simulink model "FireFighter_original"  (R2014a)
settings: Solver=ode45  StartTime=0.0  StopTime=150  RelTol=1e-3
undefined symbols (not defined in the file): DiscIntNeverNeededParam, sigbuilder_block
libraries: simulink x68
(part 3 of 6)

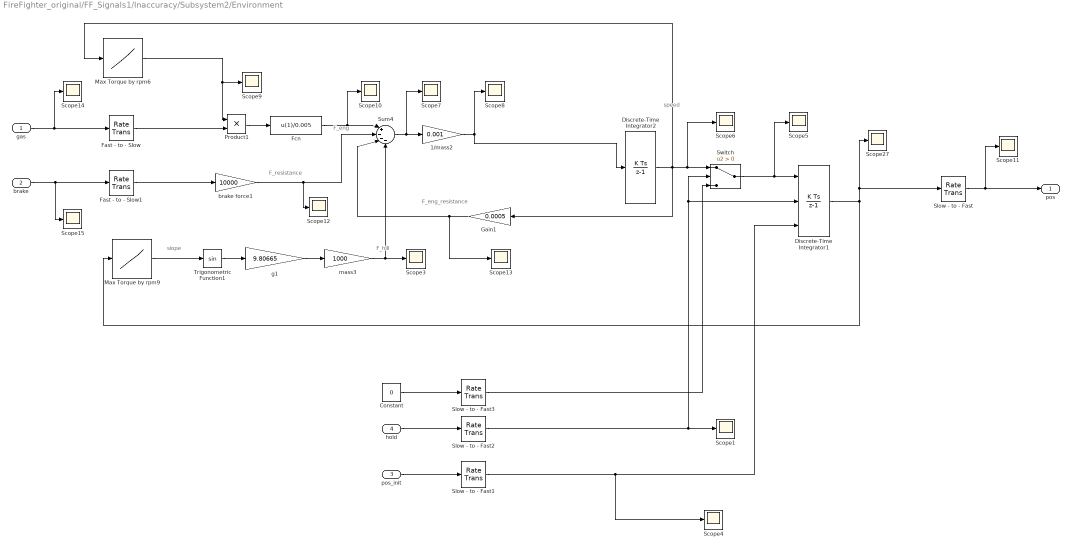
== system FireFighter_original/FF_Signals1/Inaccuracy/Subsystem2/Environment ==
  note: F_hill
  note: F_eng_resistance
  note: F_resistance
  note: F_eng
  note: speed
  note: slope
  gas : Inport
  brake : Inport  Port=2
  pos_init : Inport  Port=3
  hold : Inport  Port=4
  1/mass2 : Gain  Gain=0.001
  Constant : Constant  Value=0
  Discrete-Time Integrator1 : DiscreteIntegrator  ExternalReset=rising  InitialConditionSource=external  SampleTime=-1  ICPrevOutput=DiscIntNeverNeededParam  ICPrevScaledInput=DiscIntNeverNeededParam
  Discrete-Time Integrator2 : DiscreteIntegrator  SampleTime=-1  ICPrevOutput=DiscIntNeverNeededParam  ICPrevScaledInput=DiscIntNeverNeededParam
  Fast - to - Slow : RateTransition  OutPortSampleTimeMultiple=0.05  OutPortSampleTime=0.1
  "Fast - to - Slow1 " : RateTransition  OutPortSampleTimeMultiple=0.05  OutPortSampleTime=0.1
  Fcn : Fcn  Expr=u(1)/0.005
  Gain1 : Gain  Gain=0.0005
  Max Torque by rpm6 : Lookup_n-D  NumberOfTableDimensions=1  BreakpointsForDimension1=[0;8;20;28;40;60;80;100;120;140;160;180;200]  Table=[165;180;180;170;170;150;115;97;80;70;60;50;40]  RndMeth=Simplest  InputSameDT=on
  Max Torque by rpm9 : Lookup_n-D  NumberOfTableDimensions=1  BreakpointsForDimension1=[0:1000:15000]  Table=[0;pi/60;pi/30;pi/20;pi/15;pi/12;0;0;-pi/18;-pi/36;0;0;0;0;0;0]  RndMeth=Simplest  InputSameDT=on
  Product1 : Product  RndMeth=Zero
  Scope{1,3..15,27} (15 alike) : Scope
      Scope1 settings: TimeRange=10  YMin=-50  YMax=300  SaveName=ScopeData3
      Scope10 settings: SaveName=ScopeData23
      Scope11 settings: TimeRange=10  YMin=-50  YMax=300  SaveName=ScopeData26
      Scope12 settings: SaveName=ScopeData32
      Scope13 settings: SaveName=ScopeData33
      Scope14 settings: SaveName=ScopeData15
      Scope15 settings: SaveName=ScopeData19
      Scope27 settings: TimeRange=10  YMin=2000  YMax=3600  SaveName=ScopeData49
      Scope3 settings: SaveName=ScopeData8
      Scope4 settings: TimeRange=10  YMin=-50  YMax=300  SaveName=ScopeData13
      Scope5 settings: TimeRange=10  YMin=-50  YMax=300  SaveName=ScopeData50
      Scope6 settings: TimeRange=100  YMin=89.9904  YMax=89.9913  SaveName=ScopeData16
      Scope7 settings: SaveName=ScopeData10
      Scope8 settings: SaveName=ScopeData21
      Scope9 settings: SaveName=ScopeData22
  Slow - to - Fast{,1..3} (4 alike) : RateTransition  OutPortSampleTimeMultiple=0.05  OutPortSampleTime=0.05
  Sum4 : Sum  Inputs=|+---
  Switch : Switch  Criteria=u2 > Threshold
  Trigonometric Function1 : Trigonometry
  brake force1 : Gain  Gain=10000
  g1 : Gain  Gain=9.80665
  mass3 : Gain  Gain=1000
  pos : Outport
  wires:
  Product1/1 -> Fcn/1
  brake force1/1 -> Scope12/1, Sum4/2
  Sum4/1 -> Scope7/1, 1/mass2/1
  Gain1/1 -> Sum4/3, Scope13/1
  gas/1 -> Scope14/1, Fast - to - Slow/1
  brake/1 -> Scope15/1, "Fast - to - Slow1 "/1
  Discrete-Time Integrator2/1 -> Max Torque by rpm6/1, Scope6/1, Switch/1, Gain1/1
  Max Torque by rpm9/1 -> Trigonometric Function1/1
  g1/1 -> mass3/1
  Trigonometric Function1/1 -> g1/1
  mass3/1 -> Sum4/4, Scope3/1
  Fcn/1 -> Scope10/1, Sum4/1
  Fast - to - Slow/1 -> Product1/2
  "Fast - to - Slow1 "/1 -> brake force1/1
  Discrete-Time Integrator1/1 -> Scope27/1, Slow - to - Fast/1, Max Torque by rpm9/1
  Slow - to - Fast/1 -> pos/1, Scope11/1
  Max Torque by rpm6/1 -> Product1/1, Scope9/1
  pos_init/1 -> Slow - to - Fast1/1
  hold/1 -> Slow - to - Fast2/1
  Slow - to - Fast1/1 -> Scope4/1, Discrete-Time Integrator1/3
  Constant/1 -> Slow - to - Fast3/1
  Slow - to - Fast3/1 -> Switch/3
  Switch/1 -> Scope5/1, Discrete-Time Integrator1/1
  Slow - to - Fast2/1 -> Switch/2, Discrete-Time Integrator1/2, Scope1/1
  1/mass2/1 -> Scope8/1, Discrete-Time Integrator2/1

== system FireFighter_original/FF_Signals1/Inaccuracy/Subsystem2/FireFighter ==
  note: current speed
  note: speed=90
  pos : Inport
  Constant : Constant  Value=0
  Constant1 : Constant  Value=0
  Constant2 : Constant  Value=0
  Discrete Derivative : simulink/Discrete/Discrete Derivative  gainval=1.0  ICPrevScaledInput=0.0  InputProcessing=Inherited  OutMin=[]  OutMax=[]  OutDataType=fixdt(1, 16)  OutScaling=2^-10  DoSatur=off
  Discrete PID Controller : simulink/Continuous/PID Controller  Controller=PI  TimeDomain=Discrete-time  SampleTime=-1  IntegratorMethod=Forward Euler  FilterMethod=Forward Euler  Form=Parallel  P=0.05  I=0.000228325  D=0  N=100  InitialConditionSource=internal  InitialConditionForIntegrator=0  InitialConditionForFilter=0  ExternalReset=none  LimitOutput=on  UpperSaturationLimit=1  LowerSaturationLimit=-1  LinearizeAsGain=off  AntiWindupMode=back-calculation  Kb=0.01  TrackingMode=off  Kt=1  PParamMin=[]  PParamMax=[]  IParamMin=[]  IParamMax=[]  DParamMin=[]  DParamMax=[]  NParamMin=[]  NParamMax=[]  KbParamMin=[]  KbParamMax=[]  KtParamMin=[]  KtParamMax=[]  POutMin=[]  POutMax=[]  IOutMin=[]  IOutMax=[]  DOutMin=[]  DOutMax=[]  NOutMin=[]  NOutMax=[]  KbOutMin=[]  KbOutMax=[]  KtOutMin=[]  KtOutMax=[]  IntegratorOutMin=[]  IntegratorOutMax=[]  FilterOutMin=[]  FilterOutMax=[]  SumOutMin=[]  SumOutMax=[]  SumI1OutMin=[]  SumI1OutMax=[]  SumI2OutMin=[]  SumI2OutMax=[]  SumI3OutMin=[]  SumI3OutMax=[]  SumDOutMin=[]  SumDOutMax=[]  SaturationOutMin=[]  SaturationOutMax=[]  IntegratorContinuousStateAttributes=''  IntegratorStateMustResolveToSignalObject=off  IntegratorRTWStateStorageClass=Auto  FilterContinuousStateAttributes=''  FilterStateMustResolveToSignalObject=off  FilterRTWStateStorageClass=Auto
  Discrete PID Controller1 : simulink/Continuous/PID Controller  Controller=PI  TimeDomain=Discrete-time  SampleTime=-1  IntegratorMethod=Forward Euler  FilterMethod=Forward Euler  Form=Parallel  P=0.05  I=0.000228325  D=0  N=100  InitialConditionSource=internal  InitialConditionForIntegrator=0  InitialConditionForFilter=0  ExternalReset=none  LimitOutput=on  UpperSaturationLimit=1  LowerSaturationLimit=-1  LinearizeAsGain=off  AntiWindupMode=back-calculation  Kb=0.01  TrackingMode=off  Kt=1  PParamMin=[]  PParamMax=[]  IParamMin=[]  IParamMax=[]  DParamMin=[]  DParamMax=[]  NParamMin=[]  NParamMax=[]  KbParamMin=[]  KbParamMax=[]  KtParamMin=[]  KtParamMax=[]  POutMin=[]  POutMax=[]  IOutMin=[]  IOutMax=[]  DOutMin=[]  DOutMax=[]  NOutMin=[]  NOutMax=[]  KbOutMin=[]  KbOutMax=[]  KtOutMin=[]  KtOutMax=[]  IntegratorOutMin=[]  IntegratorOutMax=[]  FilterOutMin=[]  FilterOutMax=[]  SumOutMin=[]  SumOutMax=[]  SumI1OutMin=[]  SumI1OutMax=[]  SumI2OutMin=[]  SumI2OutMax=[]  SumI3OutMin=[]  SumI3OutMax=[]  SumDOutMin=[]  SumDOutMax=[]  SaturationOutMin=[]  SaturationOutMax=[]  IntegratorContinuousStateAttributes=''  IntegratorStateMustResolveToSignalObject=off  IntegratorRTWStateStorageClass=Auto  FilterContinuousStateAttributes=''  FilterStateMustResolveToSignalObject=off  FilterRTWStateStorageClass=Auto
  Fast - to -Slow : RateTransition  OutPortSampleTimeMultiple=0.05  OutPortSampleTime=0.1
  Fast - to -Slow1 : RateTransition  OutPortSampleTimeMultiple=0.05  OutPortSampleTime=0.1
  Fast - to -Slow2 : RateTransition  OutPortSampleTimeMultiple=0.05  OutPortSampleTime=0.1
  Gain1 : Gain  Gain=-1
  Scope{1..2,4..9,11..13} (11 alike) : Scope
      Scope1 settings: YMin=-300  YMax=300  SaveName=ScopeData52
      Scope11 settings: YMin=-300  YMax=300  SaveName=ScopeData28
      Scope12 settings: YMin=-300  YMax=300  SaveName=ScopeData30
      Scope13 settings: SaveName=ScopeData31
      Scope2 settings: YMin=-300  YMax=300  SaveName=ScopeData2
      Scope4 settings: YMin=-300  YMax=300  SaveName=ScopeData17
      Scope5 settings: SaveName=ScopeData20
      Scope6 settings: YMin=-300  YMax=300  SaveName=ScopeData18
      Scope7 settings: YMin=-300  YMax=300  SaveName=ScopeData24
      Scope8 settings: TimeRange=10  SaveName=ScopeData25
      Scope9 settings: SaveName=ScopeData38
  Slow - to - Fast : RateTransition  OutPortSampleTimeMultiple=0.05  OutPortSampleTime=0.05
  Slow - to - Fast1 : RateTransition  OutPortSampleTimeMultiple=0.05  OutPortSampleTime=0.05
  Sum : Sum  Inputs=|+-
  Switch : Switch
  Switch1 : Switch
  gas : Outport
  brake : Outport  Port=2
  wires:
  Discrete Derivative/1 -> Scope8/1, Sum/2
  Discrete PID Controller/1 -> Scope2/1, Scope7/1, Switch/1, Switch/2, Switch1/2, Gain1/1
  Gain1/1 -> Switch1/3
  Switch/1 -> Slow - to - Fast/1, Scope4/1
  Constant/1 -> Switch/3, Switch1/1
  Switch1/1 -> Slow - to - Fast1/1, Scope6/1
  pos/1 -> Scope13/1, Fast - to -Slow/1
  Sum/1 -> Discrete PID Controller/1, Scope9/1
  Fast - to -Slow/1 -> Discrete Derivative/1, Scope5/1
  Slow - to - Fast/1 -> Scope11/1, gas/1
  Slow - to - Fast1/1 -> Scope12/1, brake/1
  Constant2/1 -> Fast - to -Slow1/1
  Fast - to -Slow1/1 -> Sum/1
  Discrete PID Controller1/1 -> Scope1/1
  Constant1/1 -> Fast - to -Slow2/1
  Fast - to -Slow2/1 -> Discrete PID Controller1/1

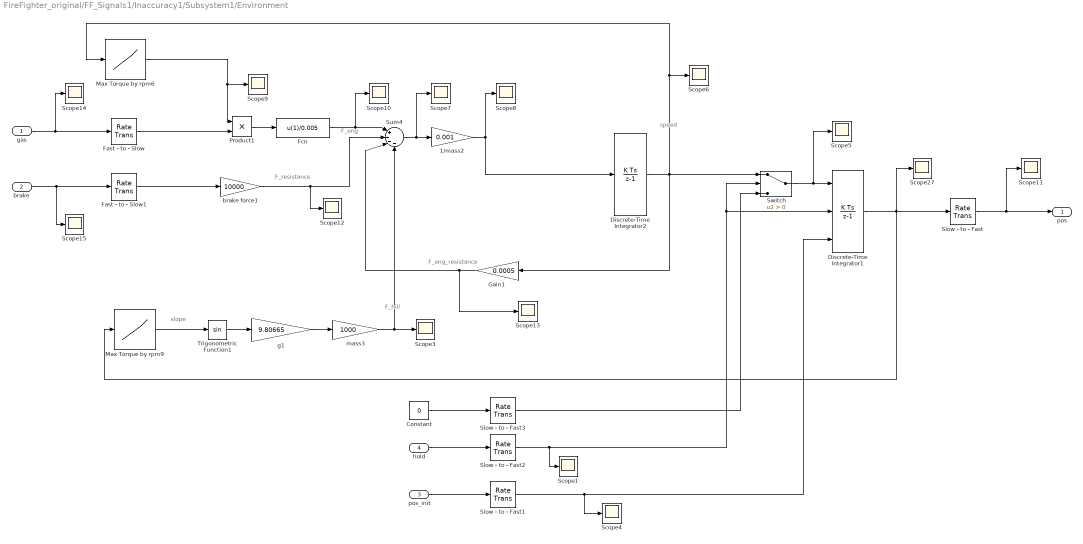
== system FireFighter_original/FF_Signals1/Inaccuracy1/Subsystem1/Environment ==
  note: F_hill
  note: F_eng_resistance
  note: F_resistance
  note: F_eng
  note: slope
  note: speed
  gas : Inport
  brake : Inport  Port=2
  pos_init : Inport  Port=3
  hold : Inport  Port=4
  1/mass2 : Gain  Gain=0.001
  Constant : Constant  Value=0
  Discrete-Time Integrator1 : DiscreteIntegrator  ExternalReset=rising  InitialConditionSource=external  SampleTime=-1  ICPrevOutput=DiscIntNeverNeededParam  ICPrevScaledInput=DiscIntNeverNeededParam
  Discrete-Time Integrator2 : DiscreteIntegrator  SampleTime=-1  ICPrevOutput=DiscIntNeverNeededParam  ICPrevScaledInput=DiscIntNeverNeededParam
  Fast - to - Slow : RateTransition  OutPortSampleTimeMultiple=0.05  OutPortSampleTime=0.1
  "Fast - to - Slow1 " : RateTransition  OutPortSampleTimeMultiple=0.05  OutPortSampleTime=0.1
  Fcn : Fcn  Expr=u(1)/0.005
  Gain1 : Gain  Gain=0.0005
  Max Torque by rpm6 : Lookup_n-D  NumberOfTableDimensions=1  BreakpointsForDimension1=[0;8;20;28;40;60;80;100;120;140;160;180;200]  Table=[165;180;180;170;170;150;115;97;80;70;60;50;40]  RndMeth=Simplest  InputSameDT=on
  Max Torque by rpm9 : Lookup_n-D  NumberOfTableDimensions=1  BreakpointsForDimension1=[0:1000:15000]  Table=[0;pi/60;pi/30;pi/20;pi/15;pi/12;0;0;-pi/18;-pi/36;0;0;0;0;0;0]  RndMeth=Simplest  InputSameDT=on
  Product1 : Product  RndMeth=Zero
  Scope{1,3..15,27} (15 alike) : Scope
      Scope1 settings: TimeRange=10  YMin=-50  YMax=300  SaveName=ScopeData51
      Scope10 settings: SaveName=ScopeData23
      Scope11 settings: TimeRange=10  YMin=-50  YMax=300  SaveName=ScopeData26
      Scope12 settings: SaveName=ScopeData32
      Scope13 settings: SaveName=ScopeData33
      Scope14 settings: SaveName=ScopeData15
      Scope15 settings: SaveName=ScopeData19
      Scope27 settings: TimeRange=10  YMin=-50  YMax=300  SaveName=ScopeData49
      Scope3 settings: SaveName=ScopeData8
      Scope4 settings: TimeRange=10  YMin=-50  YMax=300  SaveName=ScopeData53
      Scope5 settings: TimeRange=10  YMin=-50  YMax=300  SaveName=ScopeData54
      Scope6 settings: TimeRange=100  YMin=0  YMax=300  SaveName=ScopeData55
      Scope7 settings: SaveName=ScopeData10
      Scope8 settings: SaveName=ScopeData21
      Scope9 settings: SaveName=ScopeData22
  Slow - to - Fast{,1..3} (4 alike) : RateTransition  OutPortSampleTimeMultiple=0.05  OutPortSampleTime=0.05
  Sum4 : Sum  Inputs=|+---
  Switch : Switch  Criteria=u2 > Threshold
  Trigonometric Function1 : Trigonometry
  brake force1 : Gain  Gain=10000
  g1 : Gain  Gain=9.80665
  mass3 : Gain  Gain=1000
  pos : Outport
  wires:
  Product1/1 -> Fcn/1
  brake force1/1 -> Scope12/1, Sum4/2
  Sum4/1 -> Scope7/1, 1/mass2/1
  1/mass2/1 -> Discrete-Time Integrator2/1, Scope8/1
  Gain1/1 -> Scope13/1, Sum4/3
  gas/1 -> Scope14/1, Fast - to - Slow/1
  brake/1 -> Scope15/1, "Fast - to - Slow1 "/1
  Max Torque by rpm9/1 -> Trigonometric Function1/1
  g1/1 -> mass3/1
  Trigonometric Function1/1 -> g1/1
  mass3/1 -> Sum4/4, Scope3/1
  Fcn/1 -> Scope10/1, Sum4/1
  Fast - to - Slow/1 -> Product1/2
  "Fast - to - Slow1 "/1 -> brake force1/1
  Slow - to - Fast/1 -> pos/1, Scope11/1
  Max Torque by rpm6/1 -> Product1/1, Scope9/1
  Discrete-Time Integrator2/1 -> Max Torque by rpm6/1, Scope6/1, Switch/1, Gain1/1
  pos_init/1 -> Slow - to - Fast1/1
  hold/1 -> Slow - to - Fast2/1
  Slow - to - Fast2/1 -> Switch/2, Discrete-Time Integrator1/2, Scope1/1
  Slow - to - Fast1/1 -> Scope4/1, Discrete-Time Integrator1/3
  Constant/1 -> Slow - to - Fast3/1
  Slow - to - Fast3/1 -> Switch/3
  Discrete-Time Integrator1/1 -> Max Torque by rpm9/1, Scope27/1, Slow - to - Fast/1
  Switch/1 -> Scope5/1, Discrete-Time Integrator1/1

== system FireFighter_original/FF_Signals1/Inaccuracy1/Subsystem1/FireFighter ==
  note: current speed
  note: speed=90
  pos : Inport
  Constant : Constant  Value=0
  Constant1 : Constant  Value=250
  Constant2 : Constant  Value=250
  Discrete Derivative : simulink/Discrete/Discrete Derivative  gainval=1.0  ICPrevScaledInput=0.0  InputProcessing=Inherited  OutMin=[]  OutMax=[]  OutDataType=fixdt(1, 16)  OutScaling=2^-10  DoSatur=off
  Discrete PID Controller : simulink/Continuous/PID Controller  Controller=PI  TimeDomain=Discrete-time  SampleTime=-1  IntegratorMethod=Forward Euler  FilterMethod=Forward Euler  Form=Parallel  P=0.05  I=0.000228325  D=0  N=100  InitialConditionSource=internal  InitialConditionForIntegrator=0  InitialConditionForFilter=0  ExternalReset=none  LimitOutput=on  UpperSaturationLimit=1  LowerSaturationLimit=-1  LinearizeAsGain=off  AntiWindupMode=back-calculation  Kb=0.01  TrackingMode=off  Kt=1  PParamMin=[]  PParamMax=[]  IParamMin=[]  IParamMax=[]  DParamMin=[]  DParamMax=[]  NParamMin=[]  NParamMax=[]  KbParamMin=[]  KbParamMax=[]  KtParamMin=[]  KtParamMax=[]  POutMin=[]  POutMax=[]  IOutMin=[]  IOutMax=[]  DOutMin=[]  DOutMax=[]  NOutMin=[]  NOutMax=[]  KbOutMin=[]  KbOutMax=[]  KtOutMin=[]  KtOutMax=[]  IntegratorOutMin=[]  IntegratorOutMax=[]  FilterOutMin=[]  FilterOutMax=[]  SumOutMin=[]  SumOutMax=[]  SumI1OutMin=[]  SumI1OutMax=[]  SumI2OutMin=[]  SumI2OutMax=[]  SumI3OutMin=[]  SumI3OutMax=[]  SumDOutMin=[]  SumDOutMax=[]  SaturationOutMin=[]  SaturationOutMax=[]  IntegratorContinuousStateAttributes=''  IntegratorStateMustResolveToSignalObject=off  IntegratorRTWStateStorageClass=Auto  FilterContinuousStateAttributes=''  FilterStateMustResolveToSignalObject=off  FilterRTWStateStorageClass=Auto
  Discrete PID Controller1 : simulink/Continuous/PID Controller  Controller=PI  TimeDomain=Discrete-time  SampleTime=-1  IntegratorMethod=Forward Euler  FilterMethod=Forward Euler  Form=Parallel  P=0.05  I=0.000228325  D=0  N=100  InitialConditionSource=internal  InitialConditionForIntegrator=0  InitialConditionForFilter=0  ExternalReset=none  LimitOutput=on  UpperSaturationLimit=1  LowerSaturationLimit=-1  LinearizeAsGain=off  AntiWindupMode=back-calculation  Kb=0.01  TrackingMode=off  Kt=1  PParamMin=[]  PParamMax=[]  IParamMin=[]  IParamMax=[]  DParamMin=[]  DParamMax=[]  NParamMin=[]  NParamMax=[]  KbParamMin=[]  KbParamMax=[]  KtParamMin=[]  KtParamMax=[]  POutMin=[]  POutMax=[]  IOutMin=[]  IOutMax=[]  DOutMin=[]  DOutMax=[]  NOutMin=[]  NOutMax=[]  KbOutMin=[]  KbOutMax=[]  KtOutMin=[]  KtOutMax=[]  IntegratorOutMin=[]  IntegratorOutMax=[]  FilterOutMin=[]  FilterOutMax=[]  SumOutMin=[]  SumOutMax=[]  SumI1OutMin=[]  SumI1OutMax=[]  SumI2OutMin=[]  SumI2OutMax=[]  SumI3OutMin=[]  SumI3OutMax=[]  SumDOutMin=[]  SumDOutMax=[]  SaturationOutMin=[]  SaturationOutMax=[]  IntegratorContinuousStateAttributes=''  IntegratorStateMustResolveToSignalObject=off  IntegratorRTWStateStorageClass=Auto  FilterContinuousStateAttributes=''  FilterStateMustResolveToSignalObject=off  FilterRTWStateStorageClass=Auto
  Fast - to -Slow : RateTransition  OutPortSampleTimeMultiple=0.05  OutPortSampleTime=0.1
  Fast - to -Slow1 : RateTransition  OutPortSampleTimeMultiple=0.05  OutPortSampleTime=0.1
  Fast - to -Slow2 : RateTransition  OutPortSampleTimeMultiple=0.05  OutPortSampleTime=0.1
  Gain1 : Gain  Gain=-1
  Scope{1..2,4..9,11..13} (11 alike) : Scope
      Scope1 settings: YMin=-300  YMax=300  SaveName=ScopeData56
      Scope11 settings: YMin=-300  YMax=300  SaveName=ScopeData28
      Scope12 settings: YMin=-300  YMax=300  SaveName=ScopeData30
      Scope13 settings: SaveName=ScopeData31
      Scope2 settings: YMin=-300  YMax=300  SaveName=ScopeData2
      Scope4 settings: YMin=-300  YMax=300  SaveName=ScopeData17
      Scope5 settings: SaveName=ScopeData20
      Scope6 settings: YMin=-300  YMax=300  SaveName=ScopeData18
      Scope7 settings: YMin=-300  YMax=300  SaveName=ScopeData24
      Scope8 settings: TimeRange=10  YMin=-1  YMax=1  SaveName=ScopeData25
      Scope9 settings: SaveName=ScopeData38
  Slow - to - Fast : RateTransition  OutPortSampleTimeMultiple=0.05  OutPortSampleTime=0.05
  Slow - to - Fast1 : RateTransition  OutPortSampleTimeMultiple=0.05  OutPortSampleTime=0.05
  Sum : Sum  Inputs=|+-
  Switch : Switch
  Switch1 : Switch
  gas : Outport
  brake : Outport  Port=2
  wires:
  Discrete Derivative/1 -> Scope8/1, Sum/2
  Discrete PID Controller/1 -> Scope2/1, Scope7/1, Switch/1, Switch/2, Switch1/2, Gain1/1
  Gain1/1 -> Switch1/3
  Switch/1 -> Slow - to - Fast/1, Scope4/1
  Constant/1 -> Switch/3, Switch1/1
  Switch1/1 -> Slow - to - Fast1/1, Scope6/1
  pos/1 -> Scope13/1, Fast - to -Slow/1
  Sum/1 -> Discrete PID Controller/1, Scope9/1
  Fast - to -Slow/1 -> Discrete Derivative/1, Scope5/1
  Slow - to - Fast/1 -> Scope11/1, gas/1
  Slow - to - Fast1/1 -> Scope12/1, brake/1
  Constant2/1 -> Fast - to -Slow1/1
  Fast - to -Slow1/1 -> Sum/1
  Constant1/1 -> Fast - to -Slow2/1
  Fast - to -Slow2/1 -> Discrete PID Controller1/1
  Discrete PID Controller1/1 -> Scope1/1

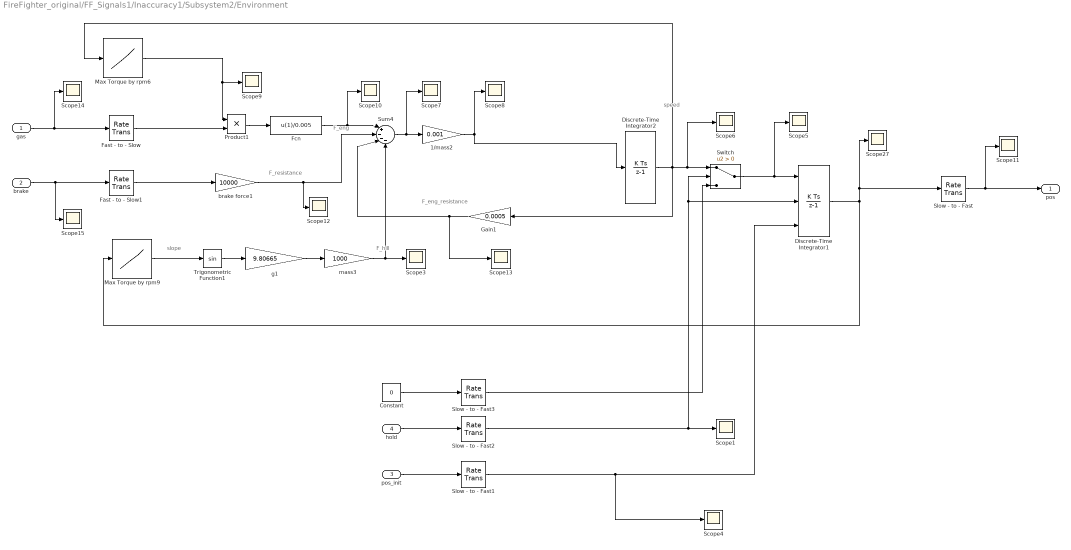
== system FireFighter_original/FF_Signals1/Inaccuracy1/Subsystem2/Environment ==
  note: F_hill
  note: F_eng_resistance
  note: F_resistance
  note: F_eng
  note: speed
  note: slope
  gas : Inport
  brake : Inport  Port=2
  pos_init : Inport  Port=3
  hold : Inport  Port=4
  1/mass2 : Gain  Gain=0.001
  Constant : Constant  Value=0
  Discrete-Time Integrator1 : DiscreteIntegrator  ExternalReset=rising  InitialConditionSource=external  SampleTime=-1  ICPrevOutput=DiscIntNeverNeededParam  ICPrevScaledInput=DiscIntNeverNeededParam
  Discrete-Time Integrator2 : DiscreteIntegrator  SampleTime=-1  ICPrevOutput=DiscIntNeverNeededParam  ICPrevScaledInput=DiscIntNeverNeededParam
  Fast - to - Slow : RateTransition  OutPortSampleTimeMultiple=0.05  OutPortSampleTime=0.1
  "Fast - to - Slow1 " : RateTransition  OutPortSampleTimeMultiple=0.05  OutPortSampleTime=0.1
  Fcn : Fcn  Expr=u(1)/0.005
  Gain1 : Gain  Gain=0.0005
  Max Torque by rpm6 : Lookup_n-D  NumberOfTableDimensions=1  BreakpointsForDimension1=[0;8;20;28;40;60;80;100;120;140;160;180;200]  Table=[165;180;180;170;170;150;115;97;80;70;60;50;40]  RndMeth=Simplest  InputSameDT=on
  Max Torque by rpm9 : Lookup_n-D  NumberOfTableDimensions=1  BreakpointsForDimension1=[0:1000:15000]  Table=[0;pi/60;pi/30;pi/20;pi/15;pi/12;0;0;-pi/18;-pi/36;0;0;0;0;0;0]  RndMeth=Simplest  InputSameDT=on
  Product1 : Product  RndMeth=Zero
  Scope{1,3..15,27} (15 alike) : Scope
      Scope1 settings: TimeRange=10  YMin=-50  YMax=300  SaveName=ScopeData3
      Scope10 settings: SaveName=ScopeData23
      Scope11 settings: TimeRange=10  YMin=-50  YMax=300  SaveName=ScopeData26
      Scope12 settings: SaveName=ScopeData32
      Scope13 settings: SaveName=ScopeData33
      Scope14 settings: SaveName=ScopeData15
      Scope15 settings: SaveName=ScopeData19
      Scope27 settings: TimeRange=10  YMin=2000  YMax=3600  SaveName=ScopeData49
      Scope3 settings: SaveName=ScopeData8
      Scope4 settings: TimeRange=10  YMin=-50  YMax=300  SaveName=ScopeData13
      Scope5 settings: TimeRange=10  YMin=-50  YMax=300  SaveName=ScopeData50
      Scope6 settings: TimeRange=100  YMin=89.9904  YMax=89.9913  SaveName=ScopeData16
      Scope7 settings: SaveName=ScopeData10
      Scope8 settings: SaveName=ScopeData21
      Scope9 settings: SaveName=ScopeData22
  Slow - to - Fast{,1..3} (4 alike) : RateTransition  OutPortSampleTimeMultiple=0.05  OutPortSampleTime=0.05
  Sum4 : Sum  Inputs=|+---
  Switch : Switch  Criteria=u2 > Threshold
  Trigonometric Function1 : Trigonometry
  brake force1 : Gain  Gain=10000
  g1 : Gain  Gain=9.80665
  mass3 : Gain  Gain=1000
  pos : Outport
  wires:
  Product1/1 -> Fcn/1
  brake force1/1 -> Scope12/1, Sum4/2
  Sum4/1 -> Scope7/1, 1/mass2/1
  Gain1/1 -> Sum4/3, Scope13/1
  gas/1 -> Scope14/1, Fast - to - Slow/1
  brake/1 -> Scope15/1, "Fast - to - Slow1 "/1
  Discrete-Time Integrator2/1 -> Max Torque by rpm6/1, Scope6/1, Switch/1, Gain1/1
  Max Torque by rpm9/1 -> Trigonometric Function1/1
  g1/1 -> mass3/1
  Trigonometric Function1/1 -> g1/1
  mass3/1 -> Sum4/4, Scope3/1
  Fcn/1 -> Scope10/1, Sum4/1
  Fast - to - Slow/1 -> Product1/2
  "Fast - to - Slow1 "/1 -> brake force1/1
  Discrete-Time Integrator1/1 -> Scope27/1, Slow - to - Fast/1, Max Torque by rpm9/1
  Slow - to - Fast/1 -> pos/1, Scope11/1
  Max Torque by rpm6/1 -> Product1/1, Scope9/1
  pos_init/1 -> Slow - to - Fast1/1
  hold/1 -> Slow - to - Fast2/1
  Slow - to - Fast1/1 -> Scope4/1, Discrete-Time Integrator1/3
  Constant/1 -> Slow - to - Fast3/1
  Slow - to - Fast3/1 -> Switch/3
  Switch/1 -> Scope5/1, Discrete-Time Integrator1/1
  Slow - to - Fast2/1 -> Switch/2, Discrete-Time Integrator1/2, Scope1/1
  1/mass2/1 -> Scope8/1, Discrete-Time Integrator2/1

== system FireFighter_original/FF_Signals1/Inaccuracy1/Subsystem2/FireFighter ==
  note: current speed
  note: speed=90
  pos : Inport
  Constant : Constant  Value=0
  Constant1 : Constant  Value=0
  Constant2 : Constant  Value=0
  Discrete Derivative : simulink/Discrete/Discrete Derivative  gainval=1.0  ICPrevScaledInput=0.0  InputProcessing=Inherited  OutMin=[]  OutMax=[]  OutDataType=fixdt(1, 16)  OutScaling=2^-10  DoSatur=off
  Discrete PID Controller : simulink/Continuous/PID Controller  Controller=PI  TimeDomain=Discrete-time  SampleTime=-1  IntegratorMethod=Forward Euler  FilterMethod=Forward Euler  Form=Parallel  P=0.05  I=0.000228325  D=0  N=100  InitialConditionSource=internal  InitialConditionForIntegrator=0  InitialConditionForFilter=0  ExternalReset=none  LimitOutput=on  UpperSaturationLimit=1  LowerSaturationLimit=-1  LinearizeAsGain=off  AntiWindupMode=back-calculation  Kb=0.01  TrackingMode=off  Kt=1  PParamMin=[]  PParamMax=[]  IParamMin=[]  IParamMax=[]  DParamMin=[]  DParamMax=[]  NParamMin=[]  NParamMax=[]  KbParamMin=[]  KbParamMax=[]  KtParamMin=[]  KtParamMax=[]  POutMin=[]  POutMax=[]  IOutMin=[]  IOutMax=[]  DOutMin=[]  DOutMax=[]  NOutMin=[]  NOutMax=[]  KbOutMin=[]  KbOutMax=[]  KtOutMin=[]  KtOutMax=[]  IntegratorOutMin=[]  IntegratorOutMax=[]  FilterOutMin=[]  FilterOutMax=[]  SumOutMin=[]  SumOutMax=[]  SumI1OutMin=[]  SumI1OutMax=[]  SumI2OutMin=[]  SumI2OutMax=[]  SumI3OutMin=[]  SumI3OutMax=[]  SumDOutMin=[]  SumDOutMax=[]  SaturationOutMin=[]  SaturationOutMax=[]  IntegratorContinuousStateAttributes=''  IntegratorStateMustResolveToSignalObject=off  IntegratorRTWStateStorageClass=Auto  FilterContinuousStateAttributes=''  FilterStateMustResolveToSignalObject=off  FilterRTWStateStorageClass=Auto
  Discrete PID Controller1 : simulink/Continuous/PID Controller  Controller=PI  TimeDomain=Discrete-time  SampleTime=-1  IntegratorMethod=Forward Euler  FilterMethod=Forward Euler  Form=Parallel  P=0.05  I=0.000228325  D=0  N=100  InitialConditionSource=internal  InitialConditionForIntegrator=0  InitialConditionForFilter=0  ExternalReset=none  LimitOutput=on  UpperSaturationLimit=1  LowerSaturationLimit=-1  LinearizeAsGain=off  AntiWindupMode=back-calculation  Kb=0.01  TrackingMode=off  Kt=1  PParamMin=[]  PParamMax=[]  IParamMin=[]  IParamMax=[]  DParamMin=[]  DParamMax=[]  NParamMin=[]  NParamMax=[]  KbParamMin=[]  KbParamMax=[]  KtParamMin=[]  KtParamMax=[]  POutMin=[]  POutMax=[]  IOutMin=[]  IOutMax=[]  DOutMin=[]  DOutMax=[]  NOutMin=[]  NOutMax=[]  KbOutMin=[]  KbOutMax=[]  KtOutMin=[]  KtOutMax=[]  IntegratorOutMin=[]  IntegratorOutMax=[]  FilterOutMin=[]  FilterOutMax=[]  SumOutMin=[]  SumOutMax=[]  SumI1OutMin=[]  SumI1OutMax=[]  SumI2OutMin=[]  SumI2OutMax=[]  SumI3OutMin=[]  SumI3OutMax=[]  SumDOutMin=[]  SumDOutMax=[]  SaturationOutMin=[]  SaturationOutMax=[]  IntegratorContinuousStateAttributes=''  IntegratorStateMustResolveToSignalObject=off  IntegratorRTWStateStorageClass=Auto  FilterContinuousStateAttributes=''  FilterStateMustResolveToSignalObject=off  FilterRTWStateStorageClass=Auto
  Fast - to -Slow : RateTransition  OutPortSampleTimeMultiple=0.05  OutPortSampleTime=0.1
  Fast - to -Slow1 : RateTransition  OutPortSampleTimeMultiple=0.05  OutPortSampleTime=0.1
  Fast - to -Slow2 : RateTransition  OutPortSampleTimeMultiple=0.05  OutPortSampleTime=0.1
  Gain1 : Gain  Gain=-1
  Scope{1..2,4..9,11..13} (11 alike) : Scope
      Scope1 settings: YMin=-300  YMax=300  SaveName=ScopeData52
      Scope11 settings: YMin=-300  YMax=300  SaveName=ScopeData28
      Scope12 settings: YMin=-300  YMax=300  SaveName=ScopeData30
      Scope13 settings: SaveName=ScopeData31
      Scope2 settings: YMin=-300  YMax=300  SaveName=ScopeData2
      Scope4 settings: YMin=-300  YMax=300  SaveName=ScopeData17
      Scope5 settings: SaveName=ScopeData20
      Scope6 settings: YMin=-300  YMax=300  SaveName=ScopeData18
      Scope7 settings: YMin=-300  YMax=300  SaveName=ScopeData24
      Scope8 settings: TimeRange=10  SaveName=ScopeData25
      Scope9 settings: SaveName=ScopeData38
  Slow - to - Fast : RateTransition  OutPortSampleTimeMultiple=0.05  OutPortSampleTime=0.05
  Slow - to - Fast1 : RateTransition  OutPortSampleTimeMultiple=0.05  OutPortSampleTime=0.05
  Sum : Sum  Inputs=|+-
  Switch : Switch
  Switch1 : Switch
  gas : Outport
  brake : Outport  Port=2
  wires:
  Discrete Derivative/1 -> Scope8/1, Sum/2
  Discrete PID Controller/1 -> Scope2/1, Scope7/1, Switch/1, Switch/2, Switch1/2, Gain1/1
  Gain1/1 -> Switch1/3
  Switch/1 -> Slow - to - Fast/1, Scope4/1
  Constant/1 -> Switch/3, Switch1/1
  Switch1/1 -> Slow - to - Fast1/1, Scope6/1
  pos/1 -> Scope13/1, Fast - to -Slow/1
  Sum/1 -> Discrete PID Controller/1, Scope9/1
  Fast - to -Slow/1 -> Discrete Derivative/1, Scope5/1
  Slow - to - Fast/1 -> Scope11/1, gas/1
  Slow - to - Fast1/1 -> Scope12/1, brake/1
  Constant2/1 -> Fast - to -Slow1/1
  Fast - to -Slow1/1 -> Sum/1
  Discrete PID Controller1/1 -> Scope1/1
  Constant1/1 -> Fast - to -Slow2/1
  Fast - to -Slow2/1 -> Discrete PID Controller1/1

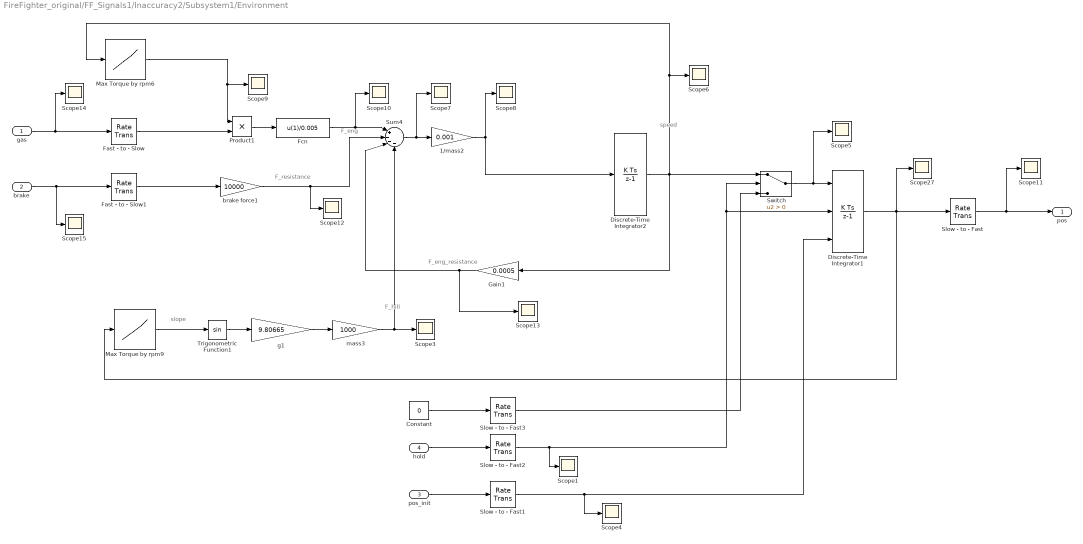
== system FireFighter_original/FF_Signals1/Inaccuracy2/Subsystem1/Environment ==
  note: F_hill
  note: F_eng_resistance
  note: F_resistance
  note: F_eng
  note: slope
  note: speed
  gas : Inport
  brake : Inport  Port=2
  pos_init : Inport  Port=3
  hold : Inport  Port=4
  1/mass2 : Gain  Gain=0.001
  Constant : Constant  Value=0
  Discrete-Time Integrator1 : DiscreteIntegrator  ExternalReset=rising  InitialConditionSource=external  SampleTime=-1  ICPrevOutput=DiscIntNeverNeededParam  ICPrevScaledInput=DiscIntNeverNeededParam
  Discrete-Time Integrator2 : DiscreteIntegrator  SampleTime=-1  ICPrevOutput=DiscIntNeverNeededParam  ICPrevScaledInput=DiscIntNeverNeededParam
  Fast - to - Slow : RateTransition  OutPortSampleTimeMultiple=0.05  OutPortSampleTime=0.1
  "Fast - to - Slow1 " : RateTransition  OutPortSampleTimeMultiple=0.05  OutPortSampleTime=0.1
  Fcn : Fcn  Expr=u(1)/0.005
  Gain1 : Gain  Gain=0.0005
  Max Torque by rpm6 : Lookup_n-D  NumberOfTableDimensions=1  BreakpointsForDimension1=[0;8;20;28;40;60;80;100;120;140;160;180;200]  Table=[165;180;180;170;170;150;115;97;80;70;60;50;40]  RndMeth=Simplest  InputSameDT=on
  Max Torque by rpm9 : Lookup_n-D  NumberOfTableDimensions=1  BreakpointsForDimension1=[0:1000:15000]  Table=[0;pi/60;pi/30;pi/20;pi/15;pi/12;0;0;-pi/18;-pi/36;0;0;0;0;0;0]  RndMeth=Simplest  InputSameDT=on
  Product1 : Product  RndMeth=Zero
  Scope{1,3..15,27} (15 alike) : Scope
      Scope1 settings: TimeRange=10  YMin=-50  YMax=300  SaveName=ScopeData51
      Scope10 settings: SaveName=ScopeData23
      Scope11 settings: TimeRange=10  YMin=-50  YMax=300  SaveName=ScopeData26
      Scope12 settings: SaveName=ScopeData32
      Scope13 settings: SaveName=ScopeData33
      Scope14 settings: SaveName=ScopeData15
      Scope15 settings: SaveName=ScopeData19
      Scope27 settings: TimeRange=10  YMin=-50  YMax=300  SaveName=ScopeData49
      Scope3 settings: SaveName=ScopeData8
      Scope4 settings: TimeRange=10  YMin=-50  YMax=300  SaveName=ScopeData53
      Scope5 settings: TimeRange=10  YMin=-50  YMax=300  SaveName=ScopeData54
      Scope6 settings: TimeRange=100  YMin=0  YMax=300  SaveName=ScopeData55
      Scope7 settings: SaveName=ScopeData10
      Scope8 settings: SaveName=ScopeData21
      Scope9 settings: SaveName=ScopeData22
  Slow - to - Fast{,1..3} (4 alike) : RateTransition  OutPortSampleTimeMultiple=0.05  OutPortSampleTime=0.05
  Sum4 : Sum  Inputs=|+---
  Switch : Switch  Criteria=u2 > Threshold
  Trigonometric Function1 : Trigonometry
  brake force1 : Gain  Gain=10000
  g1 : Gain  Gain=9.80665
  mass3 : Gain  Gain=1000
  pos : Outport
  wires:
  Product1/1 -> Fcn/1
  brake force1/1 -> Scope12/1, Sum4/2
  Sum4/1 -> Scope7/1, 1/mass2/1
  1/mass2/1 -> Discrete-Time Integrator2/1, Scope8/1
  Gain1/1 -> Scope13/1, Sum4/3
  gas/1 -> Scope14/1, Fast - to - Slow/1
  brake/1 -> Scope15/1, "Fast - to - Slow1 "/1
  Max Torque by rpm9/1 -> Trigonometric Function1/1
  g1/1 -> mass3/1
  Trigonometric Function1/1 -> g1/1
  mass3/1 -> Sum4/4, Scope3/1
  Fcn/1 -> Scope10/1, Sum4/1
  Fast - to - Slow/1 -> Product1/2
  "Fast - to - Slow1 "/1 -> brake force1/1
  Slow - to - Fast/1 -> pos/1, Scope11/1
  Max Torque by rpm6/1 -> Product1/1, Scope9/1
  Discrete-Time Integrator2/1 -> Max Torque by rpm6/1, Scope6/1, Switch/1, Gain1/1
  pos_init/1 -> Slow - to - Fast1/1
  hold/1 -> Slow - to - Fast2/1
  Slow - to - Fast2/1 -> Switch/2, Discrete-Time Integrator1/2, Scope1/1
  Slow - to - Fast1/1 -> Scope4/1, Discrete-Time Integrator1/3
  Constant/1 -> Slow - to - Fast3/1
  Slow - to - Fast3/1 -> Switch/3
  Discrete-Time Integrator1/1 -> Max Torque by rpm9/1, Scope27/1, Slow - to - Fast/1
  Switch/1 -> Scope5/1, Discrete-Time Integrator1/1

== system FireFighter_original/FF_Signals1/Inaccuracy2/Subsystem1/FireFighter ==
  note: current speed
  note: speed=90
  pos : Inport
  Constant : Constant  Value=0
  Constant1 : Constant  Value=250
  Constant2 : Constant  Value=250
  Discrete Derivative : simulink/Discrete/Discrete Derivative  gainval=1.0  ICPrevScaledInput=0.0  InputProcessing=Inherited  OutMin=[]  OutMax=[]  OutDataType=fixdt(1, 16)  OutScaling=2^-10  DoSatur=off
  Discrete PID Controller : simulink/Continuous/PID Controller  Controller=PI  TimeDomain=Discrete-time  SampleTime=-1  IntegratorMethod=Forward Euler  FilterMethod=Forward Euler  Form=Parallel  P=0.05  I=0.000228325  D=0  N=100  InitialConditionSource=internal  InitialConditionForIntegrator=0  InitialConditionForFilter=0  ExternalReset=none  LimitOutput=on  UpperSaturationLimit=1  LowerSaturationLimit=-1  LinearizeAsGain=off  AntiWindupMode=back-calculation  Kb=0.01  TrackingMode=off  Kt=1  PParamMin=[]  PParamMax=[]  IParamMin=[]  IParamMax=[]  DParamMin=[]  DParamMax=[]  NParamMin=[]  NParamMax=[]  KbParamMin=[]  KbParamMax=[]  KtParamMin=[]  KtParamMax=[]  POutMin=[]  POutMax=[]  IOutMin=[]  IOutMax=[]  DOutMin=[]  DOutMax=[]  NOutMin=[]  NOutMax=[]  KbOutMin=[]  KbOutMax=[]  KtOutMin=[]  KtOutMax=[]  IntegratorOutMin=[]  IntegratorOutMax=[]  FilterOutMin=[]  FilterOutMax=[]  SumOutMin=[]  SumOutMax=[]  SumI1OutMin=[]  SumI1OutMax=[]  SumI2OutMin=[]  SumI2OutMax=[]  SumI3OutMin=[]  SumI3OutMax=[]  SumDOutMin=[]  SumDOutMax=[]  SaturationOutMin=[]  SaturationOutMax=[]  IntegratorContinuousStateAttributes=''  IntegratorStateMustResolveToSignalObject=off  IntegratorRTWStateStorageClass=Auto  FilterContinuousStateAttributes=''  FilterStateMustResolveToSignalObject=off  FilterRTWStateStorageClass=Auto
  Discrete PID Controller1 : simulink/Continuous/PID Controller  Controller=PI  TimeDomain=Discrete-time  SampleTime=-1  IntegratorMethod=Forward Euler  FilterMethod=Forward Euler  Form=Parallel  P=0.05  I=0.000228325  D=0  N=100  InitialConditionSource=internal  InitialConditionForIntegrator=0  InitialConditionForFilter=0  ExternalReset=none  LimitOutput=on  UpperSaturationLimit=1  LowerSaturationLimit=-1  LinearizeAsGain=off  AntiWindupMode=back-calculation  Kb=0.01  TrackingMode=off  Kt=1  PParamMin=[]  PParamMax=[]  IParamMin=[]  IParamMax=[]  DParamMin=[]  DParamMax=[]  NParamMin=[]  NParamMax=[]  KbParamMin=[]  KbParamMax=[]  KtParamMin=[]  KtParamMax=[]  POutMin=[]  POutMax=[]  IOutMin=[]  IOutMax=[]  DOutMin=[]  DOutMax=[]  NOutMin=[]  NOutMax=[]  KbOutMin=[]  KbOutMax=[]  KtOutMin=[]  KtOutMax=[]  IntegratorOutMin=[]  IntegratorOutMax=[]  FilterOutMin=[]  FilterOutMax=[]  SumOutMin=[]  SumOutMax=[]  SumI1OutMin=[]  SumI1OutMax=[]  SumI2OutMin=[]  SumI2OutMax=[]  SumI3OutMin=[]  SumI3OutMax=[]  SumDOutMin=[]  SumDOutMax=[]  SaturationOutMin=[]  SaturationOutMax=[]  IntegratorContinuousStateAttributes=''  IntegratorStateMustResolveToSignalObject=off  IntegratorRTWStateStorageClass=Auto  FilterContinuousStateAttributes=''  FilterStateMustResolveToSignalObject=off  FilterRTWStateStorageClass=Auto
  Fast - to -Slow : RateTransition  OutPortSampleTimeMultiple=0.05  OutPortSampleTime=0.1
  Fast - to -Slow1 : RateTransition  OutPortSampleTimeMultiple=0.05  OutPortSampleTime=0.1
  Fast - to -Slow2 : RateTransition  OutPortSampleTimeMultiple=0.05  OutPortSampleTime=0.1
  Gain1 : Gain  Gain=-1
  Scope{1..2,4..9,11..13} (11 alike) : Scope
      Scope1 settings: YMin=-300  YMax=300  SaveName=ScopeData56
      Scope11 settings: YMin=-300  YMax=300  SaveName=ScopeData28
      Scope12 settings: YMin=-300  YMax=300  SaveName=ScopeData30
      Scope13 settings: SaveName=ScopeData31
      Scope2 settings: YMin=-300  YMax=300  SaveName=ScopeData2
      Scope4 settings: YMin=-300  YMax=300  SaveName=ScopeData17
      Scope5 settings: SaveName=ScopeData20
      Scope6 settings: YMin=-300  YMax=300  SaveName=ScopeData18
      Scope7 settings: YMin=-300  YMax=300  SaveName=ScopeData24
      Scope8 settings: TimeRange=10  YMin=-1  YMax=1  SaveName=ScopeData25
      Scope9 settings: SaveName=ScopeData38
  Slow - to - Fast : RateTransition  OutPortSampleTimeMultiple=0.05  OutPortSampleTime=0.05
  Slow - to - Fast1 : RateTransition  OutPortSampleTimeMultiple=0.05  OutPortSampleTime=0.05
  Sum : Sum  Inputs=|+-
  Switch : Switch
  Switch1 : Switch
  gas : Outport
  brake : Outport  Port=2
  wires:
  Discrete Derivative/1 -> Scope8/1, Sum/2
  Discrete PID Controller/1 -> Scope2/1, Scope7/1, Switch/1, Switch/2, Switch1/2, Gain1/1
  Gain1/1 -> Switch1/3
  Switch/1 -> Slow - to - Fast/1, Scope4/1
  Constant/1 -> Switch/3, Switch1/1
  Switch1/1 -> Slow - to - Fast1/1, Scope6/1
  pos/1 -> Scope13/1, Fast - to -Slow/1
  Sum/1 -> Discrete PID Controller/1, Scope9/1
  Fast - to -Slow/1 -> Discrete Derivative/1, Scope5/1
  Slow - to - Fast/1 -> Scope11/1, gas/1
  Slow - to - Fast1/1 -> Scope12/1, brake/1
  Constant2/1 -> Fast - to -Slow1/1
  Fast - to -Slow1/1 -> Sum/1
  Constant1/1 -> Fast - to -Slow2/1
  Fast - to -Slow2/1 -> Discrete PID Controller1/1
  Discrete PID Controller1/1 -> Scope1/1

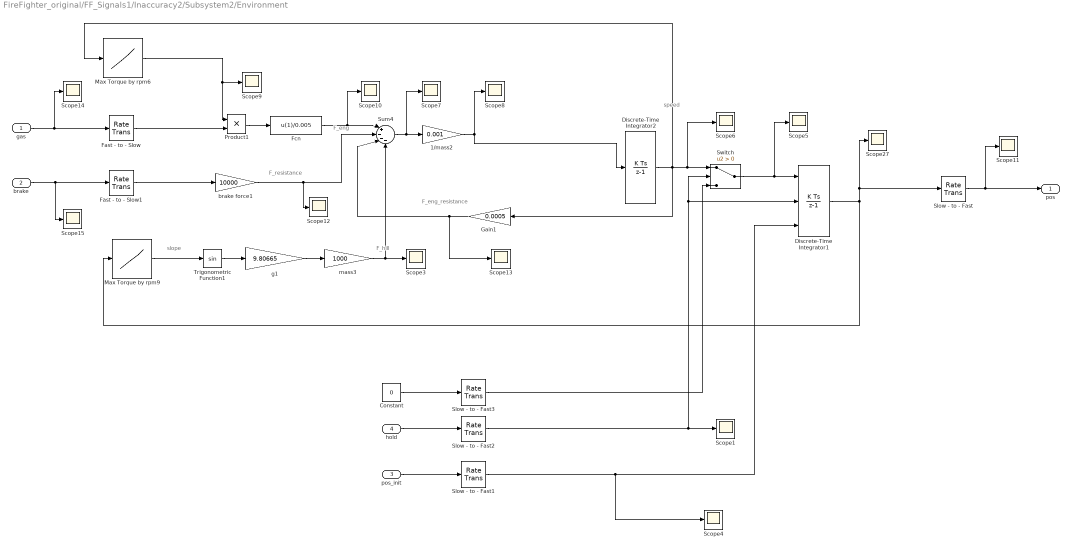
== system FireFighter_original/FF_Signals1/Inaccuracy2/Subsystem2/Environment ==
  note: F_hill
  note: F_eng_resistance
  note: F_resistance
  note: F_eng
  note: speed
  note: slope
  gas : Inport
  brake : Inport  Port=2
  pos_init : Inport  Port=3
  hold : Inport  Port=4
  1/mass2 : Gain  Gain=0.001
  Constant : Constant  Value=0
  Discrete-Time Integrator1 : DiscreteIntegrator  ExternalReset=rising  InitialConditionSource=external  SampleTime=-1  ICPrevOutput=DiscIntNeverNeededParam  ICPrevScaledInput=DiscIntNeverNeededParam
  Discrete-Time Integrator2 : DiscreteIntegrator  SampleTime=-1  ICPrevOutput=DiscIntNeverNeededParam  ICPrevScaledInput=DiscIntNeverNeededParam
  Fast - to - Slow : RateTransition  OutPortSampleTimeMultiple=0.05  OutPortSampleTime=0.1
  "Fast - to - Slow1 " : RateTransition  OutPortSampleTimeMultiple=0.05  OutPortSampleTime=0.1
  Fcn : Fcn  Expr=u(1)/0.005
  Gain1 : Gain  Gain=0.0005
  Max Torque by rpm6 : Lookup_n-D  NumberOfTableDimensions=1  BreakpointsForDimension1=[0;8;20;28;40;60;80;100;120;140;160;180;200]  Table=[165;180;180;170;170;150;115;97;80;70;60;50;40]  RndMeth=Simplest  InputSameDT=on
  Max Torque by rpm9 : Lookup_n-D  NumberOfTableDimensions=1  BreakpointsForDimension1=[0:1000:15000]  Table=[0;pi/60;pi/30;pi/20;pi/15;pi/12;0;0;-pi/18;-pi/36;0;0;0;0;0;0]  RndMeth=Simplest  InputSameDT=on
  Product1 : Product  RndMeth=Zero
  Scope{1,3..15,27} (15 alike) : Scope
      Scope1 settings: TimeRange=10  YMin=-50  YMax=300  SaveName=ScopeData3
      Scope10 settings: SaveName=ScopeData23
      Scope11 settings: TimeRange=10  YMin=-50  YMax=300  SaveName=ScopeData26
      Scope12 settings: SaveName=ScopeData32
      Scope13 settings: SaveName=ScopeData33
      Scope14 settings: SaveName=ScopeData15
      Scope15 settings: SaveName=ScopeData19
      Scope27 settings: TimeRange=10  YMin=2000  YMax=3600  SaveName=ScopeData49
      Scope3 settings: SaveName=ScopeData8
      Scope4 settings: TimeRange=10  YMin=-50  YMax=300  SaveName=ScopeData13
      Scope5 settings: TimeRange=10  YMin=-50  YMax=300  SaveName=ScopeData50
      Scope6 settings: TimeRange=100  YMin=89.9904  YMax=89.9913  SaveName=ScopeData16
      Scope7 settings: SaveName=ScopeData10
      Scope8 settings: SaveName=ScopeData21
      Scope9 settings: SaveName=ScopeData22
  Slow - to - Fast{,1..3} (4 alike) : RateTransition  OutPortSampleTimeMultiple=0.05  OutPortSampleTime=0.05
  Sum4 : Sum  Inputs=|+---
  Switch : Switch  Criteria=u2 > Threshold
  Trigonometric Function1 : Trigonometry
  brake force1 : Gain  Gain=10000
  g1 : Gain  Gain=9.80665
  mass3 : Gain  Gain=1000
  pos : Outport
  wires:
  Product1/1 -> Fcn/1
  brake force1/1 -> Scope12/1, Sum4/2
  Sum4/1 -> Scope7/1, 1/mass2/1
  Gain1/1 -> Sum4/3, Scope13/1
  gas/1 -> Scope14/1, Fast - to - Slow/1
  brake/1 -> Scope15/1, "Fast - to - Slow1 "/1
  Discrete-Time Integrator2/1 -> Max Torque by rpm6/1, Scope6/1, Switch/1, Gain1/1
  Max Torque by rpm9/1 -> Trigonometric Function1/1
  g1/1 -> mass3/1
  Trigonometric Function1/1 -> g1/1
  mass3/1 -> Sum4/4, Scope3/1
  Fcn/1 -> Scope10/1, Sum4/1
  Fast - to - Slow/1 -> Product1/2
  "Fast - to - Slow1 "/1 -> brake force1/1
  Discrete-Time Integrator1/1 -> Scope27/1, Slow - to - Fast/1, Max Torque by rpm9/1
  Slow - to - Fast/1 -> pos/1, Scope11/1
  Max Torque by rpm6/1 -> Product1/1, Scope9/1
  pos_init/1 -> Slow - to - Fast1/1
  hold/1 -> Slow - to - Fast2/1
  Slow - to - Fast1/1 -> Scope4/1, Discrete-Time Integrator1/3
  Constant/1 -> Slow - to - Fast3/1
  Slow - to - Fast3/1 -> Switch/3
  Switch/1 -> Scope5/1, Discrete-Time Integrator1/1
  Slow - to - Fast2/1 -> Switch/2, Discrete-Time Integrator1/2, Scope1/1
  1/mass2/1 -> Scope8/1, Discrete-Time Integrator2/1

== system FireFighter_original/FF_Signals1/Inaccuracy2/Subsystem2/FireFighter ==
  note: current speed
  note: speed=90
  pos : Inport
  Constant : Constant  Value=0
  Constant1 : Constant  Value=0
  Constant2 : Constant  Value=0
  Discrete Derivative : simulink/Discrete/Discrete Derivative  gainval=1.0  ICPrevScaledInput=0.0  InputProcessing=Inherited  OutMin=[]  OutMax=[]  OutDataType=fixdt(1, 16)  OutScaling=2^-10  DoSatur=off
  Discrete PID Controller : simulink/Continuous/PID Controller  Controller=PI  TimeDomain=Discrete-time  SampleTime=-1  IntegratorMethod=Forward Euler  FilterMethod=Forward Euler  Form=Parallel  P=0.05  I=0.000228325  D=0  N=100  InitialConditionSource=internal  InitialConditionForIntegrator=0  InitialConditionForFilter=0  ExternalReset=none  LimitOutput=on  UpperSaturationLimit=1  LowerSaturationLimit=-1  LinearizeAsGain=off  AntiWindupMode=back-calculation  Kb=0.01  TrackingMode=off  Kt=1  PParamMin=[]  PParamMax=[]  IParamMin=[]  IParamMax=[]  DParamMin=[]  DParamMax=[]  NParamMin=[]  NParamMax=[]  KbParamMin=[]  KbParamMax=[]  KtParamMin=[]  KtParamMax=[]  POutMin=[]  POutMax=[]  IOutMin=[]  IOutMax=[]  DOutMin=[]  DOutMax=[]  NOutMin=[]  NOutMax=[]  KbOutMin=[]  KbOutMax=[]  KtOutMin=[]  KtOutMax=[]  IntegratorOutMin=[]  IntegratorOutMax=[]  FilterOutMin=[]  FilterOutMax=[]  SumOutMin=[]  SumOutMax=[]  SumI1OutMin=[]  SumI1OutMax=[]  SumI2OutMin=[]  SumI2OutMax=[]  SumI3OutMin=[]  SumI3OutMax=[]  SumDOutMin=[]  SumDOutMax=[]  SaturationOutMin=[]  SaturationOutMax=[]  IntegratorContinuousStateAttributes=''  IntegratorStateMustResolveToSignalObject=off  IntegratorRTWStateStorageClass=Auto  FilterContinuousStateAttributes=''  FilterStateMustResolveToSignalObject=off  FilterRTWStateStorageClass=Auto
  Discrete PID Controller1 : simulink/Continuous/PID Controller  Controller=PI  TimeDomain=Discrete-time  SampleTime=-1  IntegratorMethod=Forward Euler  FilterMethod=Forward Euler  Form=Parallel  P=0.05  I=0.000228325  D=0  N=100  InitialConditionSource=internal  InitialConditionForIntegrator=0  InitialConditionForFilter=0  ExternalReset=none  LimitOutput=on  UpperSaturationLimit=1  LowerSaturationLimit=-1  LinearizeAsGain=off  AntiWindupMode=back-calculation  Kb=0.01  TrackingMode=off  Kt=1  PParamMin=[]  PParamMax=[]  IParamMin=[]  IParamMax=[]  DParamMin=[]  DParamMax=[]  NParamMin=[]  NParamMax=[]  KbParamMin=[]  KbParamMax=[]  KtParamMin=[]  KtParamMax=[]  POutMin=[]  POutMax=[]  IOutMin=[]  IOutMax=[]  DOutMin=[]  DOutMax=[]  NOutMin=[]  NOutMax=[]  KbOutMin=[]  KbOutMax=[]  KtOutMin=[]  KtOutMax=[]  IntegratorOutMin=[]  IntegratorOutMax=[]  FilterOutMin=[]  FilterOutMax=[]  SumOutMin=[]  SumOutMax=[]  SumI1OutMin=[]  SumI1OutMax=[]  SumI2OutMin=[]  SumI2OutMax=[]  SumI3OutMin=[]  SumI3OutMax=[]  SumDOutMin=[]  SumDOutMax=[]  SaturationOutMin=[]  SaturationOutMax=[]  IntegratorContinuousStateAttributes=''  IntegratorStateMustResolveToSignalObject=off  IntegratorRTWStateStorageClass=Auto  FilterContinuousStateAttributes=''  FilterStateMustResolveToSignalObject=off  FilterRTWStateStorageClass=Auto
  Fast - to -Slow : RateTransition  OutPortSampleTimeMultiple=0.05  OutPortSampleTime=0.1
  Fast - to -Slow1 : RateTransition  OutPortSampleTimeMultiple=0.05  OutPortSampleTime=0.1
  Fast - to -Slow2 : RateTransition  OutPortSampleTimeMultiple=0.05  OutPortSampleTime=0.1
  Gain1 : Gain  Gain=-1
  Scope{1..2,4..9,11..13} (11 alike) : Scope
      Scope1 settings: YMin=-300  YMax=300  SaveName=ScopeData52
      Scope11 settings: YMin=-300  YMax=300  SaveName=ScopeData28
      Scope12 settings: YMin=-300  YMax=300  SaveName=ScopeData30
      Scope13 settings: SaveName=ScopeData31
      Scope2 settings: YMin=-300  YMax=300  SaveName=ScopeData2
      Scope4 settings: YMin=-300  YMax=300  SaveName=ScopeData17
      Scope5 settings: SaveName=ScopeData20
      Scope6 settings: YMin=-300  YMax=300  SaveName=ScopeData18
      Scope7 settings: YMin=-300  YMax=300  SaveName=ScopeData24
      Scope8 settings: TimeRange=10  SaveName=ScopeData25
      Scope9 settings: SaveName=ScopeData38
  Slow - to - Fast : RateTransition  OutPortSampleTimeMultiple=0.05  OutPortSampleTime=0.05
  Slow - to - Fast1 : RateTransition  OutPortSampleTimeMultiple=0.05  OutPortSampleTime=0.05
  Sum : Sum  Inputs=|+-
  Switch : Switch
  Switch1 : Switch
  gas : Outport
  brake : Outport  Port=2
  wires:
  Discrete Derivative/1 -> Scope8/1, Sum/2
  Discrete PID Controller/1 -> Scope2/1, Scope7/1, Switch/1, Switch/2, Switch1/2, Gain1/1
  Gain1/1 -> Switch1/3
  Switch/1 -> Slow - to - Fast/1, Scope4/1
  Constant/1 -> Switch/3, Switch1/1
  Switch1/1 -> Slow - to - Fast1/1, Scope6/1
  pos/1 -> Scope13/1, Fast - to -Slow/1
  Sum/1 -> Discrete PID Controller/1, Scope9/1
  Fast - to -Slow/1 -> Discrete Derivative/1, Scope5/1
  Slow - to - Fast/1 -> Scope11/1, gas/1
  Slow - to - Fast1/1 -> Scope12/1, brake/1
  Constant2/1 -> Fast - to -Slow1/1
  Fast - to -Slow1/1 -> Sum/1
  Discrete PID Controller1/1 -> Scope1/1
  Constant1/1 -> Fast - to -Slow2/1
  Fast - to -Slow2/1 -> Discrete PID Controller1/1

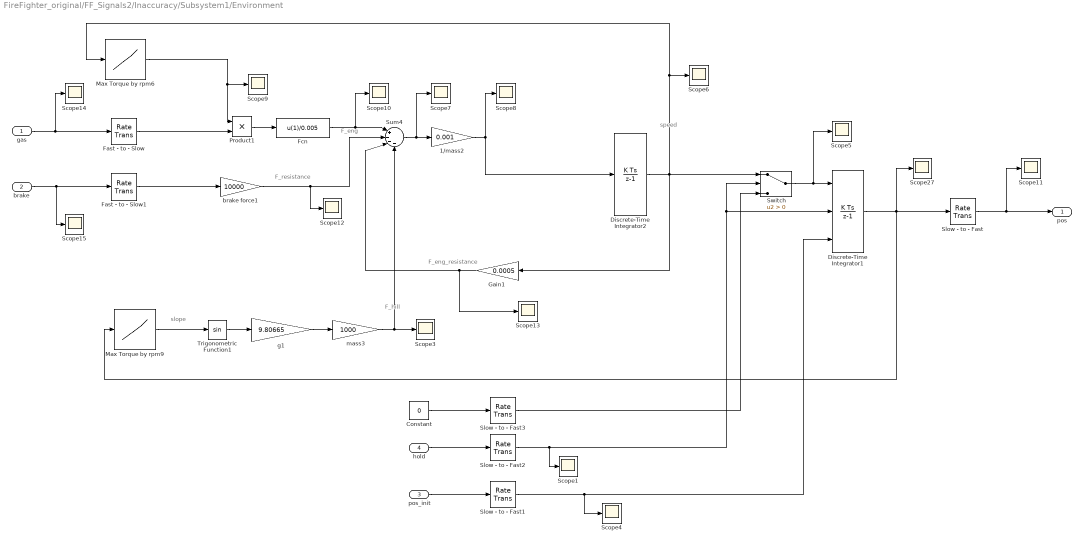
== system FireFighter_original/FF_Signals2/Inaccuracy/Subsystem1/Environment ==
  note: F_hill
  note: F_eng_resistance
  note: F_resistance
  note: F_eng
  note: slope
  note: speed
  gas : Inport
  brake : Inport  Port=2
  pos_init : Inport  Port=3
  hold : Inport  Port=4
  1/mass2 : Gain  Gain=0.001
  Constant : Constant  Value=0
  Discrete-Time Integrator1 : DiscreteIntegrator  ExternalReset=rising  InitialConditionSource=external  SampleTime=-1  ICPrevOutput=DiscIntNeverNeededParam  ICPrevScaledInput=DiscIntNeverNeededParam
  Discrete-Time Integrator2 : DiscreteIntegrator  SampleTime=-1  ICPrevOutput=DiscIntNeverNeededParam  ICPrevScaledInput=DiscIntNeverNeededParam
  Fast - to - Slow : RateTransition  OutPortSampleTimeMultiple=0.05  OutPortSampleTime=0.1
  "Fast - to - Slow1 " : RateTransition  OutPortSampleTimeMultiple=0.05  OutPortSampleTime=0.1
  Fcn : Fcn  Expr=u(1)/0.005
  Gain1 : Gain  Gain=0.0005
  Max Torque by rpm6 : Lookup_n-D  NumberOfTableDimensions=1  BreakpointsForDimension1=[0;8;20;28;40;60;80;100;120;140;160;180;200]  Table=[165;180;180;170;170;150;115;97;80;70;60;50;40]  RndMeth=Simplest  InputSameDT=on
  Max Torque by rpm9 : Lookup_n-D  NumberOfTableDimensions=1  BreakpointsForDimension1=[0:1000:15000]  Table=[0;pi/60;pi/30;pi/20;pi/15;pi/12;0;0;-pi/18;-pi/36;0;0;0;0;0;0]  RndMeth=Simplest  InputSameDT=on
  Product1 : Product  RndMeth=Zero
  Scope{1,3..15,27} (15 alike) : Scope
      Scope1 settings: TimeRange=10  YMin=-50  YMax=300  SaveName=ScopeData51
      Scope10 settings: SaveName=ScopeData23
      Scope11 settings: TimeRange=10  YMin=-50  YMax=300  SaveName=ScopeData26
      Scope12 settings: SaveName=ScopeData32
      Scope13 settings: SaveName=ScopeData33
      Scope14 settings: SaveName=ScopeData15
      Scope15 settings: SaveName=ScopeData19
      Scope27 settings: TimeRange=10  YMin=-50  YMax=300  SaveName=ScopeData49
      Scope3 settings: SaveName=ScopeData8
      Scope4 settings: TimeRange=10  YMin=-50  YMax=300  SaveName=ScopeData53
      Scope5 settings: TimeRange=10  YMin=-50  YMax=300  SaveName=ScopeData54
      Scope6 settings: TimeRange=100  YMin=0  YMax=300  SaveName=ScopeData55
      Scope7 settings: SaveName=ScopeData10
      Scope8 settings: SaveName=ScopeData21
      Scope9 settings: SaveName=ScopeData22
  Slow - to - Fast{,1..3} (4 alike) : RateTransition  OutPortSampleTimeMultiple=0.05  OutPortSampleTime=0.05
  Sum4 : Sum  Inputs=|+---
  Switch : Switch  Criteria=u2 > Threshold
  Trigonometric Function1 : Trigonometry
  brake force1 : Gain  Gain=10000
  g1 : Gain  Gain=9.80665
  mass3 : Gain  Gain=1000
  pos : Outport
  wires:
  Product1/1 -> Fcn/1
  brake force1/1 -> Scope12/1, Sum4/2
  Sum4/1 -> Scope7/1, 1/mass2/1
  1/mass2/1 -> Discrete-Time Integrator2/1, Scope8/1
  Gain1/1 -> Scope13/1, Sum4/3
  gas/1 -> Scope14/1, Fast - to - Slow/1
  brake/1 -> Scope15/1, "Fast - to - Slow1 "/1
  Max Torque by rpm9/1 -> Trigonometric Function1/1
  g1/1 -> mass3/1
  Trigonometric Function1/1 -> g1/1
  mass3/1 -> Sum4/4, Scope3/1
  Fcn/1 -> Scope10/1, Sum4/1
  Fast - to - Slow/1 -> Product1/2
  "Fast - to - Slow1 "/1 -> brake force1/1
  Slow - to - Fast/1 -> pos/1, Scope11/1
  Max Torque by rpm6/1 -> Product1/1, Scope9/1
  Discrete-Time Integrator2/1 -> Max Torque by rpm6/1, Scope6/1, Switch/1, Gain1/1
  pos_init/1 -> Slow - to - Fast1/1
  hold/1 -> Slow - to - Fast2/1
  Slow - to - Fast2/1 -> Switch/2, Discrete-Time Integrator1/2, Scope1/1
  Slow - to - Fast1/1 -> Scope4/1, Discrete-Time Integrator1/3
  Constant/1 -> Slow - to - Fast3/1
  Slow - to - Fast3/1 -> Switch/3
  Discrete-Time Integrator1/1 -> Max Torque by rpm9/1, Scope27/1, Slow - to - Fast/1
  Switch/1 -> Scope5/1, Discrete-Time Integrator1/1
